simulink model "FAST"  (R2016a)
settings: Solver=FixedStepAuto  SolverMode=SingleTasking  StartTime=0.0  StopTime=600  FixedStep=DT  RelTol=1e-3
values from neighbouring files (symbols this model uses):
  delta_1p = (25*pi)/180    (= 0.436332312999)    [IPC_Control.m]
  delta_2p = (33*pi)/180    (= 0.575958653158)    [IPC_Control.m]
  IPC_Pitch_max = 5    [IPC_Control.m]
  k_1p = 1E-3    (= 0.001)    [IPC_Control.m]
  k_2p = 1E-3    (= 0.001)    [IPC_Control.m]
  ki_1p = 0.01    [IPC_Control.m]
  ki_2p = 0.002    [IPC_Control.m]
  omega_1p = (2*pi)/4.95    (= 1.26933036509)    [IPC_Control.m]
  omega_2p = (4*pi)/4.95    (= 2.53866073017)    [IPC_Control.m]
  omega_L = 10    [IPC_Control.m]
  zeta_1p = 0.5    [IPC_Control.m]
  zeta_2p = 0.3    [IPC_Control.m]
  zeta_L = 1    [IPC_Control.m]
undefined symbols (not defined in the file or in its folder): CertificationSettings, Control, DiscIntNeverNeededParam, dLP, Drivetrain, OutList, P_InitAngle, RPM_Init, strmatch, T_GenSpeedInit
settings Model: ExtModeTrigMode=oneshot  ExtModeArmWhenConnect=off  Creator=Hazim Namik  LastModifiedBy=jwvanwingerden
settings DataIOCC: LimitDataPoints=on  SaveFormat=Array
settings OptimizationCC: BlockReduction=off  BooleanDataType=off
settings DebuggingCC: SaveWithParameterizedLinksMsg=none  UnderspecifiedInitializationDetection=Classic  MergeDetectMultiDrivingBlocksExec=none  SignalResolutionControl=TryResolveAllWithWarning
settings HardwareCC: ProdBitPerPointer=32  ProdLargestAtomicFloat=None  ProdIntDivRoundTo=Undefined  ProdEndianess=Unspecified  ProdWordSize=32  ProdHWDeviceType=32-bit Generic  TargetUnknown=on
settings ModelReferenceCC: PropagateSignalLabelsOutOfModel=off

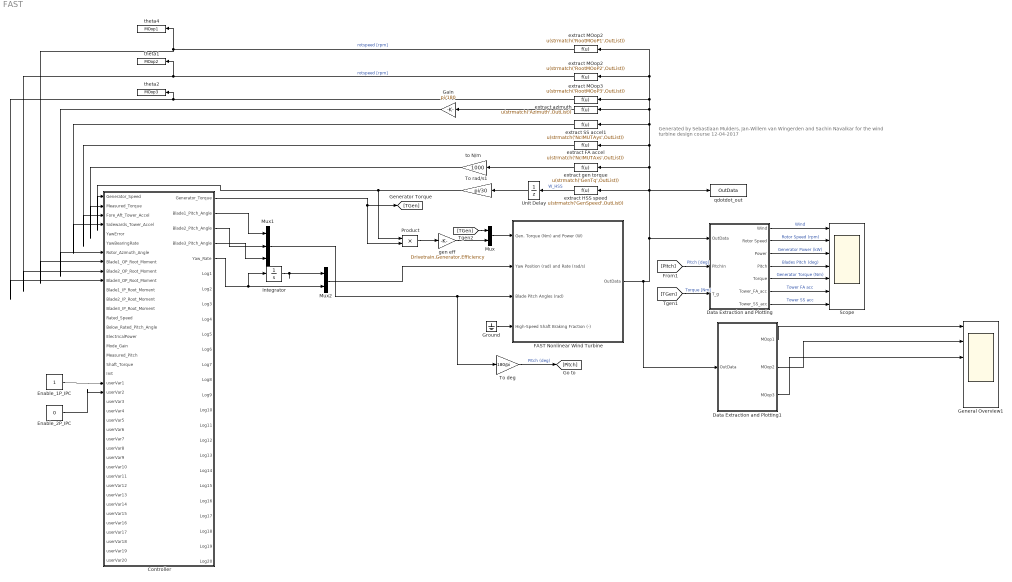
== system FAST ==
  note: Generated by Sebastiaan Mulders, Jan-Willem van Wingerden and Sachin Navalkar
      | for the wind turbine design course 12-04-2017
  Controller : Subsystem
  Data Extraction and Plotting : Subsystem
  Data Extraction and Plotting1 : Subsystem
  Enable_1P_IPC : Constant
  Enable_2P_IPC : Constant  Value=0
  FAST Nonlinear Wind Turbine : Subsystem  mask(FAST Nonlinear Wind Turbine){}
      mask help: This block contains the FAST S-Function.
      mask init:
      | clear FAST_SFunc
  Gain : Gain  Gain=pi/180
  General Overview1 : Scope  NumInputPorts=6
  Ground : Ground
  Integrator : Integrator
  Mux : Mux  Inputs=2
  Mux1 : Mux  Inputs=3
  Mux2 : Mux  Inputs=2
  Product : Product  RndMeth=Zero
  Scope : Scope  NumInputPorts=7
      settings: Tag=Scope
  To deg : Gain  Gain=180/pi
  To rad/s1 : Gain  Gain=pi/30
  Unit Delay : UnitDelay  InitialCondition=RPM_Init*Drivetrain.Gearbox.Ratio  SampleTime=-1
  extract FA accel : Fcn  Expr=u(strmatch('NcIMUTAxs',OutList))
  extract HSS speed : Fcn  Expr=u(strmatch('GenSpeed',OutList))
  extract MOop2 : Fcn  Expr=u(strmatch('RootMOoP2',OutList))
  "extract MOop2 " : Fcn  Expr=u(strmatch('RootMOoP1',OutList))
  extract MOop3 : Fcn  Expr=u(strmatch('RootMOoP3',OutList))
  extract SS accel1 : Fcn  Expr=u(strmatch('NcIMUTAys',OutList))
  extract azimuth : Fcn  Expr=u(strmatch('Azimuth',OutList))
  extract gen torque : Fcn  Expr=u(strmatch('GenTq',OutList))
  gen eff : Gain  Gain=Drivetrain.Generator.Efficiency
  qdotdot_out : ToWorkspace  VariableName=OutData  SampleTime=-1
  theta1 : ToWorkspace  VariableName=MOop2
      settings: MaxDataPoints=Inf
  theta2 : ToWorkspace  VariableName=MOop3
      settings: MaxDataPoints=Inf
  theta4 : ToWorkspace  VariableName=MOop1
      settings: MaxDataPoints=Inf
  to N/m : Gain  Gain=1000
  wires:
  Mux/1 -> FAST Nonlinear Wind Turbine/1(Gen. Torque (Nm) and Power (W))
  Mux2/1 -> FAST Nonlinear Wind Turbine/2(Yaw Position (rad) and Rate (rad/s))
  extract HSS speed/1 -> Unit Delay/1  "W_HSS"
  To deg/1 -> [Pitch]  "Pitch (deg)"
  gen eff/1 -> Mux/2
  Product/1 -> gen eff/1
  To rad/s1/1 -> Product/1, Controller/1(Generator_Speed)
  Data Extraction and Plotting/3(Power) -> Scope/3  "Generator Power (kW)"
  [Pitch] -> Data Extraction and Plotting/2(PitchIn)  "Pitch [deg]"
  Data Extraction and Plotting/1(Wind) -> Scope/1  "Wind"
  Data Extraction and Plotting/2(Rotor Speed) -> Scope/2  "Rotor Speed (rpm)"
  [TGen] -> Data Extraction and Plotting/3(T_g)  "Torque [Nm]"
  FAST Nonlinear Wind Turbine/1(OutData) -> Data Extraction and Plotting1/1(OutData), extract azimuth/1, extract MOop3/1, extract MOop2/1, "extract MOop2 "/1, extract SS accel1/1, extract FA accel/1, extract gen torque/1, extract HSS speed/1, qdotdot_out/1, Data Extraction and Plotting/1(OutData)
  Data Extraction and Plotting/4(Pitch) -> Scope/4  "Blades Pitch (deg)"
  Data Extraction and Plotting/5(Torque) -> Scope/5  "Generator Torque (Nm)"
  Unit Delay/1 -> To rad/s1/1
  extract gen torque/1 -> to N/m/1
  to N/m/1 -> Controller/2(Measured_Torque)
  Controller/1(Generator_Torque) -> Product/2, [TGen]
  extract FA accel/1 -> Controller/3(Fore_Aft_Tower_Accel)
  Data Extraction and Plotting/6(Tower_FA_acc) -> Scope/6  "Tower FA acc"
  Data Extraction and Plotting/7(Tower_SS_acc) -> Scope/7  "Tower SS acc"
  Ground/1 -> FAST Nonlinear Wind Turbine/4(High-Speed Shaft Braking Fraction (-))
  [TGen] -> Mux/1
  Mux1/1 -> To deg/1, FAST Nonlinear Wind Turbine/3(Blade Pitch Angles (rad))
  extract SS accel1/1 -> Controller/4(Sidewards_Tower_Accel)
  Controller/2(Blade1_Pitch_Angle) -> Mux1/1
  Controller/3(Blade2_Pitch_Angle) -> Mux1/2
  Controller/4(Blade3_Pitch_Angle) -> Mux1/3
  Integrator/1 -> Mux2/1
  Controller/5(Yaw_Rate) -> Integrator/1, Mux2/2
  "extract MOop2 "/1 -> theta4/1, Controller/8(Blade1_OP_Root_Moment)  "rotspeed [rpm]"
  extract MOop2/1 -> theta1/1, Controller/9(Blade2_OP_Root_Moment)  "rotspeed [rpm]"
  extract MOop3/1 -> Controller/10(Blade3_OP_Root_Moment), theta2/1
  Enable_1P_IPC/1 -> Controller/21(userVar1)
  Enable_2P_IPC/1 -> Controller/22(userVar2)
  extract azimuth/1 -> Gain/1
  Gain/1 -> Controller/7(Rotor_Azimuth_Angle)
  Data Extraction and Plotting1/1(MOop1) -> General Overview1/1
  Data Extraction and Plotting1/2(MOop2) -> General Overview1/2
  Data Extraction and Plotting1/3(MOop3) -> General Overview1/3

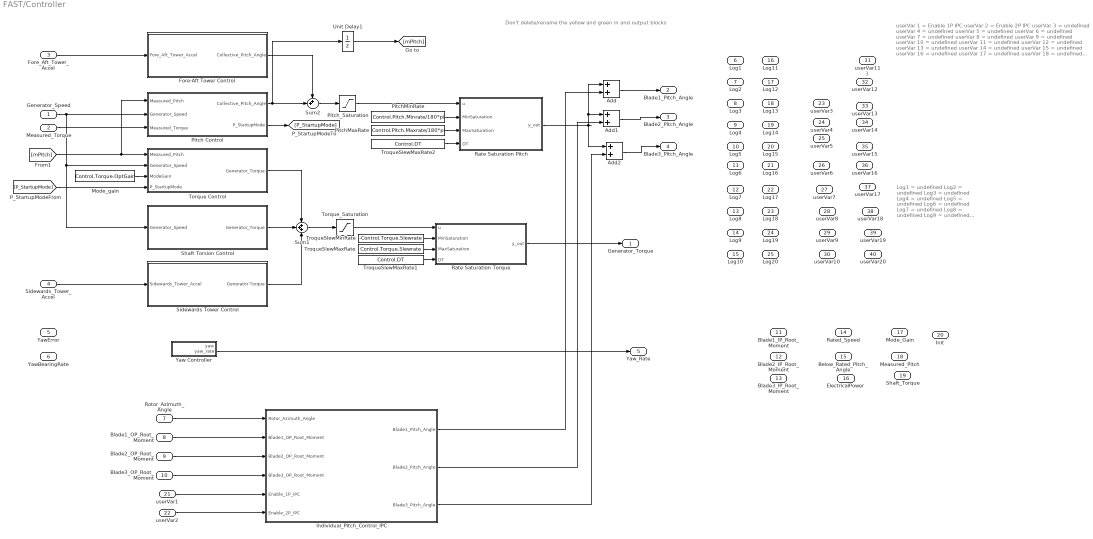
== system FAST/Controller ==
  note: Log1 		= 	undefined
      | Log2 		= 	undefined
      | Log3 		= 	undefined
      | Log4 		= 	undefined
      | Log5 		= 	undefined
      | Log6 		= 	undefined
      | Log7 		= 	undefined
      | Log8 		= 	undefined
      | Log9 		= 	undefined
      | Log10 		= 	undefined
      | Log11 		= 	undefined
      | Log12 		= 	undefined
      | Log13 		= 	undefined
      | Log14 		= 	undefined
      | Log15 		= 	undefined
      | Log16 		= 	undefined
      | Log17 		= 	undefined
      | Log18 		= 	undefined
      | Log19 		= 	undefined
      | Log20 		= 	undefined
  note: userVar 1 	=	Enable 1P IPC
      | userVar 2 	=	Enable 2P IPC
      | userVar 3 	=	undefined
      | userVar 4 	=	undefined
      | userVar 5 	=	undefined
      | userVar 6 	=	undefined
      | userVar 7 	=	undefined
      | userVar 8 	=	undefined
      | userVar 9 	=	undefined
      | userVar 10 	=	undefined
      | userVar 11 	=	undefined
      | userVar 12 	=	undefined
      | userVar 13 	=	undefined
      | userVar 14 	=	undefined
      | userVar 15 	=	undefined
      | userVar 16 	=	undefined
      | userVar 17 	=	undefined
      | userVar 18 	=	undefined
      | userVar 19 	=	undefined
      | userVar 20 	=	undefined
  note: Don't delete/rename the yellow and green in and output blocks
  note: 3
  Generator_Speed : Inport
  Measured_Torque : Inport  Port=2
  Fore_Aft_Tower_Accel : Inport  Port=3
  Sidewards_Tower_Accel : Inport  Port=4  PortDimensions=1
  YawError : Inport  Port=5  PortDimensions=1
  YawBearingRate : Inport  Port=6  PortDimensions=1
  Rotor_Azimuth_Angle : Inport  Port=7  PortDimensions=1
  Blade1_OP_Root_Moment : Inport  Port=8  PortDimensions=1
  Blade2_OP_Root_Moment : Inport  Port=9  PortDimensions=1
  Blade3_OP_Root_Moment : Inport  Port=10  PortDimensions=1
  Blade1_IP_Root_Moment : Inport  Port=11  PortDimensions=1
  Blade2_IP_Root_Moment : Inport  Port=12  PortDimensions=1
  Blade3_IP_Root_Moment : Inport  Port=13  PortDimensions=1
  Rated_Speed : Inport  Port=14  PortDimensions=1
  Below_Rated_Pitch_Angle : Inport  Port=15  PortDimensions=1
  ElectricalPower : Inport  Port=16  PortDimensions=1
  Mode_Gain : Inport  Port=17  PortDimensions=1
  Measured_Pitch : Inport  Port=18  PortDimensions=1
  Shaft_Torque : Inport  Port=19  PortDimensions=1
  Init : Inport  Port=20  PortDimensions=1
  userVar1 : Inport  Port=21  PortDimensions=1
  userVar2 : Inport  Port=22  PortDimensions=1
  userVar3 : Inport  Port=23  PortDimensions=1
  userVar4 : Inport  Port=24  PortDimensions=1
  userVar5 : Inport  Port=25  PortDimensions=1
  userVar6 : Inport  Port=26  PortDimensions=1
  userVar7 : Inport  Port=27  PortDimensions=1
  userVar8 : Inport  Port=28  PortDimensions=1
  userVar9 : Inport  Port=29  PortDimensions=1
  userVar10 : Inport  Port=30  PortDimensions=1
  userVar11 : Inport  Port=31  PortDimensions=1
  userVar12 : Inport  Port=32  PortDimensions=1
  userVar13 : Inport  Port=33  PortDimensions=1
  userVar14 : Inport  Port=34  PortDimensions=1
  userVar15 : Inport  Port=35  PortDimensions=1
  userVar16 : Inport  Port=36  PortDimensions=1
  userVar17 : Inport  Port=37  PortDimensions=1
  userVar18 : Inport  Port=38  PortDimensions=1
  userVar19 : Inport  Port=39  PortDimensions=1
  userVar20 : Inport  Port=40  PortDimensions=1
  Add : Sum
  Add1 : Sum
  Add2 : Sum
  Fore-Aft Tower Control : Subsystem
  Individual_Pitch_Control_IPC : Subsystem
  Mode_gain : Constant  Value=Control.Torque.OptGain
  Pitch Control : Subsystem
  PitchMaxRate : Constant  Value=Control.Pitch.Maxrate/180*pi
  PitchMinRate : Constant  Value=Control.Pitch.Minrate/180*pi
  Pitch_Saturation : Saturate  UpperLimit=Control.Pitch.Max*pi/180  LowerLimit=Control.Pitch.Min*pi/180
  Rate Saturation Pitch : MATLAB Function  TreatAsAtomicUnit=on
  Rate Saturation Torque : MATLAB Function  TreatAsAtomicUnit=on
  Shaft Torsion Control : Subsystem
  Sidewards Tower Control : Subsystem
  Sum1 : Sum  Inputs=+++
  Sum2 : Sum  Inputs=++|
  Torque Control : Subsystem
  Torque_Saturation : Saturate  UpperLimit=Control.Torque.Limit  LowerLimit=Control.Torque.Min
  TroqueSlewMaxRate : Constant  Value=Control.Torque.Slewrate
  TroqueSlewMaxRate1 : Constant  Value=Control.DT
  TroqueSlewMaxRate2 : Constant  Value=Control.DT
  TroqueSlewMinRate : Constant  Value=-Control.Torque.Slewrate
  Unit Delay1 : UnitDelay  InitialCondition=P_InitAngle*pi/180  SampleTime=-1
  Yaw Controller : Subsystem
  Generator_Torque : Outport
  Blade1_Pitch_Angle : Outport  Port=2  PortDimensions=1
  Blade2_Pitch_Angle : Outport  Port=3  PortDimensions=1
  Blade3_Pitch_Angle : Outport  Port=4  PortDimensions=1
  Yaw_Rate : Outport  Port=5  PortDimensions=1
  Log1 : Outport  Port=6  PortDimensions=1
  Log2 : Outport  Port=7  PortDimensions=1
  Log3 : Outport  Port=8  PortDimensions=1
  Log4 : Outport  Port=9  PortDimensions=1
  Log5 : Outport  Port=10  PortDimensions=1
  Log6 : Outport  Port=11  PortDimensions=1
  Log7 : Outport  Port=12  PortDimensions=1
  Log8 : Outport  Port=13  PortDimensions=1
  Log9 : Outport  Port=14  PortDimensions=1
  Log10 : Outport  Port=15  PortDimensions=1
  Log11 : Outport  Port=16  PortDimensions=1
  Log12 : Outport  Port=17  PortDimensions=1
  Log13 : Outport  Port=18  PortDimensions=1
  Log14 : Outport  Port=19  PortDimensions=1
  Log15 : Outport  Port=20  PortDimensions=1
  Log16 : Outport  Port=21  PortDimensions=1
  Log17 : Outport  Port=22  PortDimensions=1
  Log18 : Outport  Port=23  PortDimensions=1
  Log19 : Outport  Port=24  PortDimensions=1
  Log20 : Outport  Port=25  PortDimensions=1
  wires:
  Sidewards_Tower_Accel/1 -> Sidewards Tower Control/1(Sidewards_Tower_Accel)
  Fore_Aft_Tower_Accel/1 -> Fore-Aft Tower Control/1(Fore_Aft_Tower_Accel)
  Fore-Aft Tower Control/1(Collective_Pitch_Angle) -> Sum2/1
  Torque Control/1(Generator_Torque) -> Sum1/1
  Sidewards Tower Control/1(Generator Torque) -> Sum1/3
  [mPitch] -> Pitch Control/1(Measured_Pitch), Torque Control/1(Measured_Pitch)
  Measured_Torque/1 -> Pitch Control/3(Measured_Torque)
  Shaft Torsion Control/1(Generator_Torque) -> Sum1/2
  Mode_gain/1 -> Torque Control/3(ModeGain)
  Sum1/1 -> Torque_Saturation/1
  Unit Delay1/1 -> [mPitch]
  Sum2/1 -> Pitch_Saturation/1
  PitchMinRate/1 -> Rate Saturation Pitch/2(MinSaturation)
  PitchMaxRate/1 -> Rate Saturation Pitch/3(MaxSaturation)
  Pitch_Saturation/1 -> Rate Saturation Pitch/1(u)
  Torque_Saturation/1 -> Rate Saturation Torque/1(u)
  TroqueSlewMinRate/1 -> Rate Saturation Torque/2(MinSaturation)
  TroqueSlewMaxRate/1 -> Rate Saturation Torque/3(MaxSaturation)
  Generator_Speed/1 -> Pitch Control/2(Generator_Speed), Torque Control/2(Generator_Speed), Shaft Torsion Control/1(Generator_Speed)
  [P_StartupMode] -> Torque Control/4(P_StartupMode)
  Pitch Control/2(P_StartupMode) -> [P_StartupMode]
  Pitch Control/1(Collective_Pitch_Angle) -> Sum2/2, Unit Delay1/1
  Rate Saturation Torque/1(y_out) -> Generator_Torque/1
  TroqueSlewMaxRate1/1 -> Rate Saturation Torque/4(DT)
  TroqueSlewMaxRate2/1 -> Rate Saturation Pitch/4(DT)
  Rate Saturation Pitch/1(y_out) -> Add2/1, Add1/1, Add/1
  Yaw Controller/2(yaw_rate) -> Yaw_Rate/1
  Rotor_Azimuth_Angle/1 -> Individual_Pitch_Control_IPC/1(Rotor_Azimuth_Angle)
  Blade1_OP_Root_Moment/1 -> Individual_Pitch_Control_IPC/2(Blade1_OP_Root_Moment)
  Blade2_OP_Root_Moment/1 -> Individual_Pitch_Control_IPC/3(Blade2_OP_Root_Moment)
  Blade3_OP_Root_Moment/1 -> Individual_Pitch_Control_IPC/4(Blade3_OP_Root_Moment)
  userVar1/1 -> Individual_Pitch_Control_IPC/5(Enable_1P_IPC)
  userVar2/1 -> Individual_Pitch_Control_IPC/6(Enable_2P_IPC)
  Add/1 -> Blade1_Pitch_Angle/1
  Add1/1 -> Blade2_Pitch_Angle/1
  Add2/1 -> Blade3_Pitch_Angle/1
  Individual_Pitch_Control_IPC/1(Blade1_Pitch_Angle) -> Add/2
  Individual_Pitch_Control_IPC/2(Blade2_Pitch_Angle) -> Add1/2
  Individual_Pitch_Control_IPC/3(Blade3_Pitch_Angle) -> Add2/2

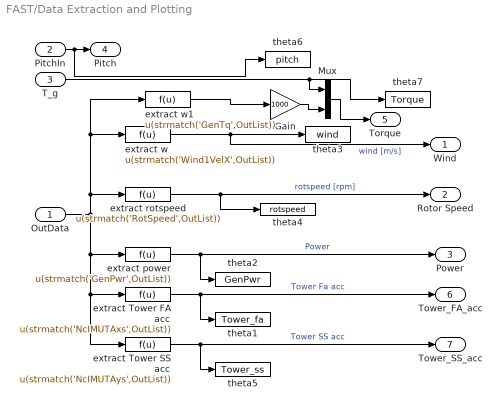
== system FAST/Data Extraction and Plotting ==
  OutData : Inport
  PitchIn : Inport  Port=2
  T_g : Inport  Port=3
  Gain : Gain  Gain=1000
  Mux : Mux  Inputs=2
  extract Tower FA acc : Fcn  Expr=u(strmatch('NcIMUTAxs',OutList))
  extract Tower SS acc : Fcn  Expr=u(strmatch('NcIMUTAys',OutList))
  extract power : Fcn  Expr=u(strmatch('GenPwr',OutList))
  extract rotspeed : Fcn  Expr=u(strmatch('RotSpeed',OutList))
  extract w : Fcn  Expr=u(strmatch('Wind1VelX',OutList))
  extract w1 : Fcn  Expr=u(strmatch('GenTq',OutList))
  theta1 : ToWorkspace  VariableName=Tower_fa  SampleTime=-1
      settings: MaxDataPoints=Inf  Decimation=3
  theta2 : ToWorkspace  VariableName=GenPwr  SampleTime=-1
      settings: MaxDataPoints=Inf  Decimation=3
  theta3 : ToWorkspace  VariableName=wind  SampleTime=-1
      settings: MaxDataPoints=Inf  Decimation=3
  theta4 : ToWorkspace  VariableName=rotspeed  SampleTime=-1
      settings: MaxDataPoints=Inf  Decimation=3
  theta5 : ToWorkspace  VariableName=Tower_ss  SampleTime=-1
      settings: MaxDataPoints=Inf  Decimation=3
  theta6 : ToWorkspace  VariableName=pitch  SampleTime=-1
      settings: MaxDataPoints=Inf  Decimation=3
  theta7 : ToWorkspace  VariableName=Torque  SampleTime=-1
      settings: MaxDataPoints=Inf  Decimation=3
  Wind : Outport
  Rotor Speed : Outport  Port=2
  Power : Outport  Port=3
  Pitch : Outport  Port=4
  Torque : Outport  Port=5
  Tower_FA_acc : Outport  Port=6
  Tower_SS_acc : Outport  Port=7
  wires:
  extract w/1 -> Wind/1, theta3/1  "wind [m/s]"
  extract rotspeed/1 -> theta4/1, Rotor Speed/1  "rotspeed [rpm]"
  extract power/1 -> theta2/1, Power/1  "Power"
  PitchIn/1 -> theta6/1, Pitch/1
  T_g/1 -> Mux/1, theta7/1
  extract Tower FA acc/1 -> theta1/1, Tower_FA_acc/1  "Tower Fa acc"
  OutData/1 -> extract w/1, extract w1/1, extract rotspeed/1, extract Tower SS acc/1, extract Tower FA acc/1, extract power/1
  extract Tower SS acc/1 -> theta5/1, Tower_SS_acc/1  "Tower SS acc"
  extract w1/1 -> Gain/1
  Gain/1 -> Mux/2
  Mux/1 -> Torque/1

== system FAST/Data Extraction and Plotting1 ==
  OutData : Inport
  "extract " : Fcn  Expr=u(strmatch('RootMOoP1',OutList))
  extract rotspeed1 : Fcn  Expr=u(strmatch('RootMOoP2',OutList))
  extract rotspeed2 : Fcn  Expr=u(strmatch('RootMOoP3',OutList))
  MOop1 : Outport
  MOop2 : Outport  Port=2
  MOop3 : Outport  Port=3
  wires:
  "extract "/1 -> MOop1/1  "rotspeed [rpm]"
  extract rotspeed1/1 -> MOop2/1  "rotspeed [rpm]"
  extract rotspeed2/1 -> MOop3/1  "rotspeed [rpm]"
  OutData/1 -> "extract "/1, extract rotspeed2/1, extract rotspeed1/1

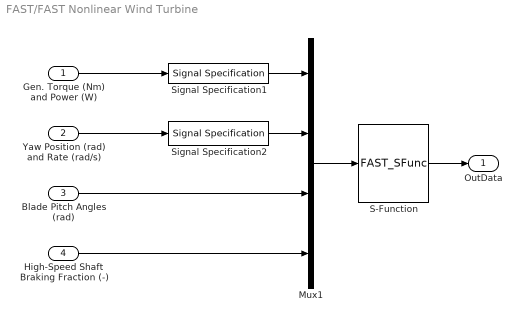
== system FAST/FAST Nonlinear Wind Turbine ==
  Gen. Torque (Nm) and Power (W) : Inport
  Yaw Position (rad) and Rate (rad/s) : Inport  Port=2
  Blade Pitch Angles (rad) : Inport  Port=3
  High-Speed Shaft Braking Fraction (-) : Inport  Port=4
  Mux1 : Mux
  S-Function : S-Function  FunctionName=FAST_SFunc  Parameters=FAST_InputFileName, TMax, 0  SFunctionDeploymentMode=off  EnableBusSupport=off
  Signal Specification1 : SignalSpecification  OutDataTypeStr=double  Dimensions=2
  Signal Specification2 : SignalSpecification  OutDataTypeStr=double  Dimensions=2
  OutData : Outport
  wires:
  Gen. Torque (Nm) and Power (W)/1 -> Signal Specification1/1
  S-Function/1 -> OutData/1
  Mux1/1 -> S-Function/1
  Blade Pitch Angles (rad)/1 -> Mux1/3
  Yaw Position (rad) and Rate (rad/s)/1 -> Signal Specification2/1
  Signal Specification1/1 -> Mux1/1
  Signal Specification2/1 -> Mux1/2
  High-Speed Shaft Braking Fraction (-)/1 -> Mux1/4

== system FAST/Controller/Fore-Aft Tower Control ==
  note: Fore-Aft tower damping
  Fore_Aft_Tower_Accel : Inport
  Discrete-Time Integrator : DiscreteIntegrator  SampleTime=-1  ICPrevOutput=DiscIntNeverNeededParam  ICPrevScaledInput=DiscIntNeverNeededParam
  Gain : Gain  Gain=Control.ForeAft.Gain
  Pitch_Saturation : Saturate  UpperLimit=Control.ForeAft.MaxPitchAmplitude*pi/180  LowerLimit=-Control.ForeAft.MaxPitchAmplitude*pi/180
  Collective_Pitch_Angle : Outport
  wires:
  Fore_Aft_Tower_Accel/1 -> Discrete-Time Integrator/1
  Pitch_Saturation/1 -> Collective_Pitch_Angle/1
  Discrete-Time Integrator/1 -> Gain/1
  Gain/1 -> Pitch_Saturation/1

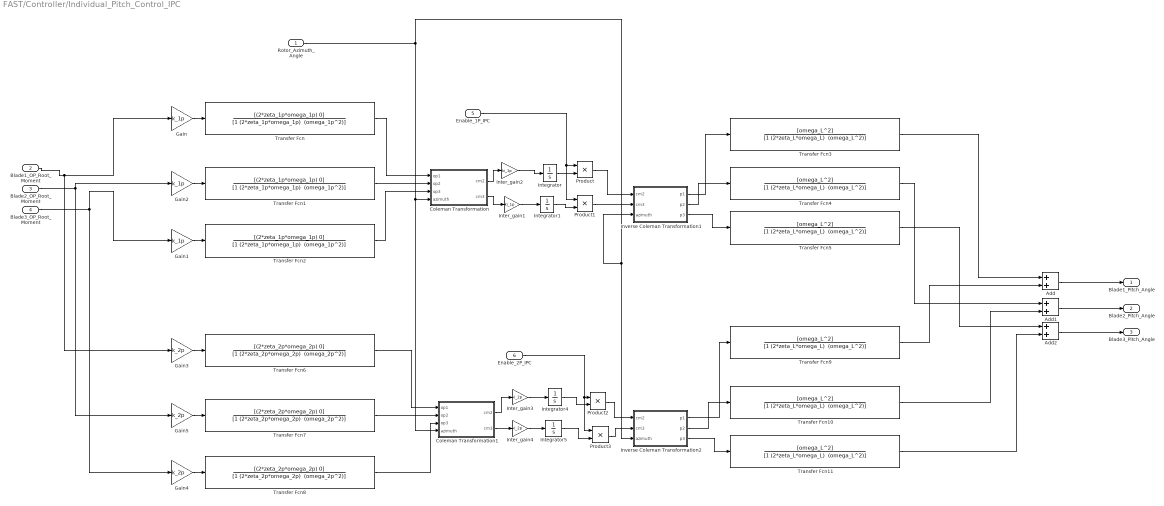
== system FAST/Controller/Individual_Pitch_Control_IPC ==
  Rotor_Azimuth_Angle : Inport
  Blade1_OP_Root_Moment : Inport  Port=2  PortDimensions=1
  Blade2_OP_Root_Moment : Inport  Port=3  PortDimensions=1
  Blade3_OP_Root_Moment : Inport  Port=4  PortDimensions=1
  Enable_1P_IPC : Inport  Port=5  PortDimensions=1
  Enable_2P_IPC : Inport  Port=6  PortDimensions=1
  Add : Sum
  Add1 : Sum
  Add2 : Sum
  Coleman Transformation : Subsystem
  Coleman Transformation1 : Subsystem
  Gain : Gain  Gain=k_1p
  Gain1 : Gain  Gain=k_1p
  Gain2 : Gain  Gain=k_1p
  Gain3 : Gain  Gain=k_2p
  Gain4 : Gain  Gain=k_2p
  Gain5 : Gain  Gain=k_2p
  Integrator{,1,4..5} (4 alike) : Integrator  LimitOutput=on  UpperSaturationLimit=IPC_Pitch_max*pi/180  LowerSaturationLimit=-IPC_Pitch_max*pi/180
  Inter_gain1 : Gain  Gain=ki_1p
  Inter_gain2 : Gain  Gain=ki_1p
  Inter_gain3 : Gain  Gain=ki_2p
  Inter_gain4 : Gain  Gain=ki_2p
  Inverse Coleman Transformation1 : Subsystem
  Inverse Coleman Transformation2 : Subsystem
  Product{,1..3} (4 alike) : Product
  Transfer Fcn : TransferFcn  Numerator=[(2*zeta_1p*omega_1p) 0]  Denominator="[1 (2*zeta_1p*omega_1p)  (omega_1p^2)]"
  Transfer Fcn1 : TransferFcn  Numerator=[(2*zeta_1p*omega_1p) 0]  Denominator="[1 (2*zeta_1p*omega_1p)  (omega_1p^2)]"
  Transfer Fcn{3..5,9..11} (6 alike) : TransferFcn  Numerator=[omega_L^2]  Denominator="[1 (2*zeta_L*omega_L)  (omega_L^2)]"
  Transfer Fcn2 : TransferFcn  Numerator=[(2*zeta_1p*omega_1p) 0]  Denominator="[1 (2*zeta_1p*omega_1p)  (omega_1p^2)]"
  Transfer Fcn6 : TransferFcn  Numerator=[(2*zeta_2p*omega_2p) 0]  Denominator="[1 (2*zeta_2p*omega_2p)  (omega_2p^2)]"
  Transfer Fcn7 : TransferFcn  Numerator=[(2*zeta_2p*omega_2p) 0]  Denominator="[1 (2*zeta_2p*omega_2p)  (omega_2p^2)]"
  Transfer Fcn8 : TransferFcn  Numerator=[(2*zeta_2p*omega_2p) 0]  Denominator="[1 (2*zeta_2p*omega_2p)  (omega_2p^2)]"
  Blade1_Pitch_Angle : Outport  PortDimensions=1
  Blade2_Pitch_Angle : Outport  Port=2  PortDimensions=1
  Blade3_Pitch_Angle : Outport  Port=3  PortDimensions=1
  wires:
  Rotor_Azimuth_Angle/1 -> Inverse Coleman Transformation1/3(azimuth), Inverse Coleman Transformation2/3(azimuth), Coleman Transformation1/4(azimuth), Coleman Transformation/4(azimuth)
  Coleman Transformation/1(cm2) -> Inter_gain2/1
  Coleman Transformation/2(cm3) -> Inter_gain1/1
  Inter_gain1/1 -> Integrator1/1
  Gain/1 -> Transfer Fcn/1
  Transfer Fcn/1 -> Coleman Transformation/1(op1)
  Gain1/1 -> Transfer Fcn2/1
  Transfer Fcn2/1 -> Coleman Transformation/3(op3)
  Gain2/1 -> Transfer Fcn1/1
  Transfer Fcn1/1 -> Coleman Transformation/2(op2)
  Inverse Coleman Transformation1/1(p1) -> Transfer Fcn3/1
  Inverse Coleman Transformation1/2(p2) -> Transfer Fcn4/1
  Inverse Coleman Transformation1/3(p3) -> Transfer Fcn5/1
  Blade1_OP_Root_Moment/1 -> Gain3/1, Gain/1
  Blade3_OP_Root_Moment/1 -> Gain1/1, Gain4/1
  Blade2_OP_Root_Moment/1 -> Gain2/1, Gain5/1
  Gain3/1 -> Transfer Fcn6/1
  Gain4/1 -> Transfer Fcn8/1
  Gain5/1 -> Transfer Fcn7/1
  Transfer Fcn6/1 -> Coleman Transformation1/1(op1)
  Transfer Fcn7/1 -> Coleman Transformation1/2(op2)
  Transfer Fcn8/1 -> Coleman Transformation1/3(op3)
  Coleman Transformation1/1(cm2) -> Inter_gain3/1
  Coleman Transformation1/2(cm3) -> Inter_gain4/1
  Inverse Coleman Transformation2/1(p1) -> Transfer Fcn9/1
  Inverse Coleman Transformation2/2(p2) -> Transfer Fcn10/1
  Inverse Coleman Transformation2/3(p3) -> Transfer Fcn11/1
  Transfer Fcn4/1 -> Add1/1
  Transfer Fcn5/1 -> Add2/1
  Transfer Fcn9/1 -> Add/2
  Transfer Fcn10/1 -> Add1/2
  Transfer Fcn11/1 -> Add2/2
  Add/1 -> Blade1_Pitch_Angle/1
  Add1/1 -> Blade2_Pitch_Angle/1
  Add2/1 -> Blade3_Pitch_Angle/1
  Inter_gain2/1 -> Integrator/1
  Transfer Fcn3/1 -> Add/1
  Inter_gain3/1 -> Integrator4/1
  Inter_gain4/1 -> Integrator5/1
  Integrator/1 -> Product/2
  Product/1 -> Inverse Coleman Transformation1/1(cm2)
  Enable_1P_IPC/1 -> Product1/1, Product/1
  Integrator1/1 -> Product1/2
  Product1/1 -> Inverse Coleman Transformation1/2(cm3)
  Enable_2P_IPC/1 -> Product3/1, Product2/1
  Integrator4/1 -> Product2/2
  Product2/1 -> Inverse Coleman Transformation2/1(cm2)
  Integrator5/1 -> Product3/2
  Product3/1 -> Inverse Coleman Transformation2/2(cm3)

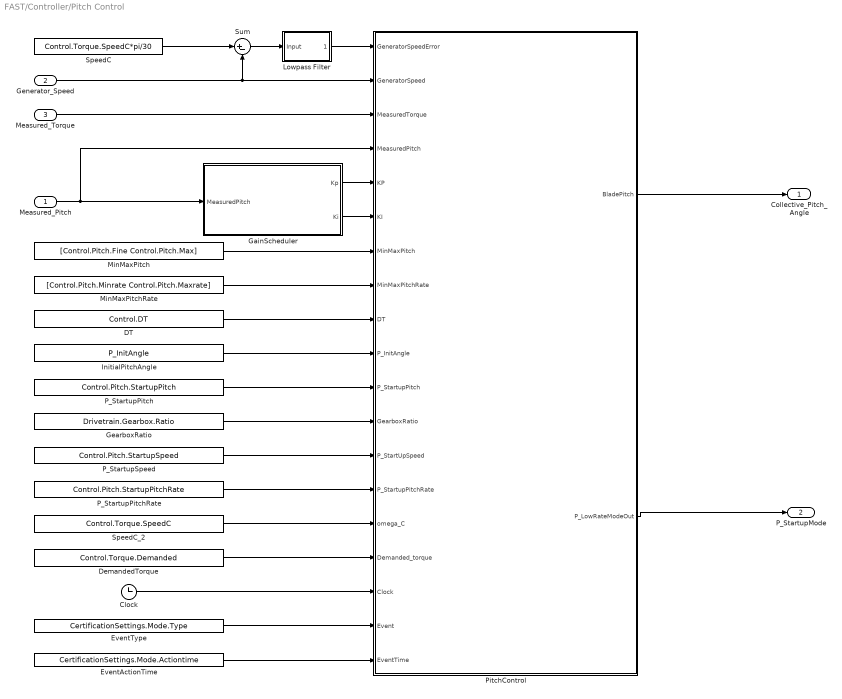
== system FAST/Controller/Pitch Control ==
  Measured_Pitch : Inport
  Generator_Speed : Inport  Port=2
  Measured_Torque : Inport  Port=3
  Clock : Clock
  DT : Constant  Value=Control.DT
  DemandedTorque : Constant  Value=Control.Torque.Demanded
  EventActionTime : Constant  Value=CertificationSettings.Mode.Actiontime
  EventType : Constant  Value=CertificationSettings.Mode.Type
  GainScheduler : Subsystem
  GearboxRatio : Constant  Value=Drivetrain.Gearbox.Ratio
  InitialPitchAngle : Constant  Value=P_InitAngle
  Lowpass Filter : Subsystem
  MinMaxPitch : Constant  Value=[Control.Pitch.Fine Control.Pitch.Max]
  MinMaxPitchRate : Constant  Value=[Control.Pitch.Minrate Control.Pitch.Maxrate]
  P_StartupPitch : Constant  Value=Control.Pitch.StartupPitch
  P_StartupPitchRate : Constant  Value=Control.Pitch.StartupPitchRate
  P_StartupSpeed : Constant  Value=Control.Pitch.StartupSpeed
  PitchControl : MATLAB Function  TreatAsAtomicUnit=on
  SpeedC : Constant  Value=Control.Torque.SpeedC*pi/30
  SpeedC_2 : Constant  Value=Control.Torque.SpeedC
  Sum : Sum  Inputs=|+-
  Collective_Pitch_Angle : Outport
  P_StartupMode : Outport  Port=2
  wires:
  MinMaxPitch/1 -> PitchControl/7(MinMaxPitch)
  MinMaxPitchRate/1 -> PitchControl/8(MinMaxPitchRate)
  PitchControl/1(BladePitch) -> Collective_Pitch_Angle/1
  Measured_Torque/1 -> PitchControl/3(MeasuredTorque)
  SpeedC/1 -> Sum/1
  Generator_Speed/1 -> PitchControl/2(GeneratorSpeed), Sum/2
  Sum/1 -> Lowpass Filter/1(Input)
  Lowpass Filter/1(Output) -> PitchControl/1(GeneratorSpeedError)
  PitchControl/2(P_LowRateModeOut) -> P_StartupMode/1
  DT/1 -> PitchControl/9(DT)
  P_StartupPitch/1 -> PitchControl/11(P_StartupPitch)
  InitialPitchAngle/1 -> PitchControl/10(P_InitAngle)
  GearboxRatio/1 -> PitchControl/12(GearboxRatio)
  P_StartupSpeed/1 -> PitchControl/13(P_StartUpSpeed)
  P_StartupPitchRate/1 -> PitchControl/14(P_StartupPitchRate)
  SpeedC_2/1 -> PitchControl/15(omega_C)
  DemandedTorque/1 -> PitchControl/16(Demanded_torque)
  Measured_Pitch/1 -> PitchControl/4(MeasuredPitch), GainScheduler/1(MeasuredPitch)
  EventType/1 -> PitchControl/18(Event)
  Clock/1 -> PitchControl/17(Clock)
  EventActionTime/1 -> PitchControl/19(EventTime)
  GainScheduler/1(Kp) -> PitchControl/5(KP)
  GainScheduler/2(Ki) -> PitchControl/6(KI)

== system FAST/Controller/Shaft Torsion Control ==
  Generator_Speed : Inport
  Gain : Gain  Gain=0
  Generator_Torque : Outport
  wires:
  Generator_Speed/1 -> Gain/1
  Gain/1 -> Generator_Torque/1

== system FAST/Controller/Sidewards Tower Control ==
  Sidewards_Tower_Accel : Inport
  Gain : Gain  Gain=0
  Generator Torque : Outport
  wires:
  Sidewards_Tower_Accel/1 -> Gain/1
  Gain/1 -> Generator Torque/1

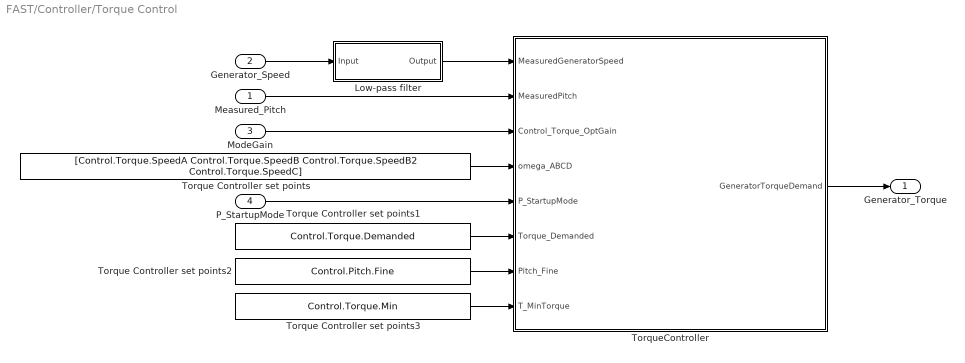
== system FAST/Controller/Torque Control ==
  Measured_Pitch : Inport
  Generator_Speed : Inport  Port=2
  ModeGain : Inport  Port=3
  P_StartupMode : Inport  Port=4
  Low-pass filter : Subsystem
  Torque Controller set points : Constant  Value=[Control.Torque.SpeedA Control.Torque.SpeedB Control.Torque.SpeedB2 Control.Torque.SpeedC]
  Torque Controller set points1 : Constant  Value=Control.Torque.Demanded
  Torque Controller set points2 : Constant  Value=Control.Pitch.Fine
  Torque Controller set points3 : Constant  Value=Control.Torque.Min
  TorqueController : MATLAB Function  TreatAsAtomicUnit=on
  Generator_Torque : Outport
  wires:
  Generator_Speed/1 -> Low-pass filter/1(Input)
  TorqueController/1(GeneratorTorqueDemand) -> Generator_Torque/1
  Measured_Pitch/1 -> TorqueController/2(MeasuredPitch)
  ModeGain/1 -> TorqueController/3(Control_Torque_OptGain)
  Torque Controller set points/1 -> TorqueController/4(omega_ABCD)
  P_StartupMode/1 -> TorqueController/5(P_StartupMode)
  Low-pass filter/1(Output) -> TorqueController/1(MeasuredGeneratorSpeed)
  Torque Controller set points3/1 -> TorqueController/8(T_MinTorque)
  Torque Controller set points2/1 -> TorqueController/7(Pitch_Fine)
  Torque Controller set points1/1 -> TorqueController/6(Torque_Demanded)

== system FAST/Controller/Yaw Controller ==
  Yaw Position : Constant  Value=0
  Yaw rate : Constant  Value=0
  yaw : Outport
  yaw_rate : Outport  Port=2
  wires:
  Yaw Position/1 -> yaw/1
  Yaw rate/1 -> yaw_rate/1

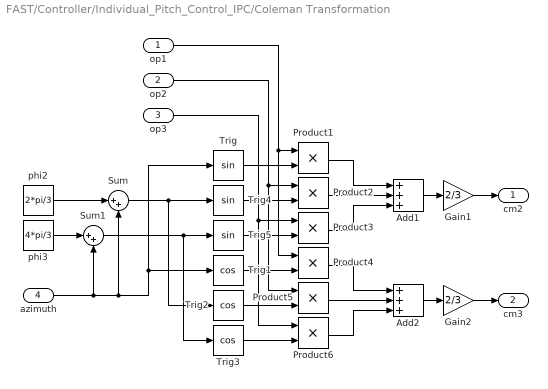
== system FAST/Controller/Individual_Pitch_Control_IPC/Coleman Transformation ==
  op1 : Inport
  op2 : Inport  Port=2
  op3 : Inport  Port=3
  azimuth : Inport  Port=4
  Add1 : Sum  Inputs=+++
  Add2 : Sum  Inputs=+++
  Gain1 : Gain  Gain=2/3
  Gain2 : Gain  Gain=2/3
  Product{1..6} (6 alike) : Product  RndMeth=Zero
  Sum : Sum  Inputs=|++
  Sum1 : Sum  Inputs=|++
  Trig : Trigonometry
  Trig1 : Trigonometry  Operator=cos
  Trig2 : Trigonometry  Operator=cos
  Trig3 : Trigonometry  Operator=cos
  Trig4 : Trigonometry
  Trig5 : Trigonometry
  phi2 : Constant  Value=2*pi/3
  phi3 : Constant  Value=4*pi/3
  cm2 : Outport
  cm3 : Outport  Port=2
  wires:
  Add1/1 -> Gain1/1
  phi2/1 -> Sum/1
  phi3/1 -> Sum1/1
  azimuth/1 -> Sum1/2, Sum/2, Trig/1, Trig1/1
  Trig/1 -> Product1/2
  Trig4/1 -> Product2/2
  Trig5/1 -> Product3/2
  Trig1/1 -> Product4/2
  Trig2/1 -> Product5/2
  Trig3/1 -> Product6/2
  Sum/1 -> Trig4/1, Trig2/1
  Sum1/1 -> Trig5/1, Trig3/1
  Add2/1 -> Gain2/1
  Gain1/1 -> cm2/1
  Gain2/1 -> cm3/1
  op1/1 -> Product1/1, Product4/1
  op2/1 -> Product2/1, Product5/1
  op3/1 -> Product6/1, Product3/1
  Product1/1 -> Add1/1
  Product2/1 -> Add1/2
  Product3/1 -> Add1/3
  Product4/1 -> Add2/1
  Product5/1 -> Add2/2
  Product6/1 -> Add2/3

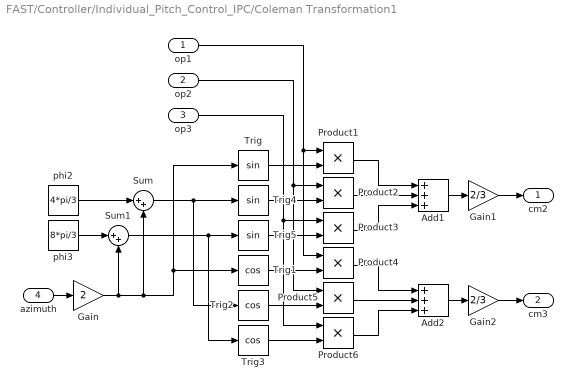
== system FAST/Controller/Individual_Pitch_Control_IPC/Coleman Transformation1 ==
  op1 : Inport
  op2 : Inport  Port=2
  op3 : Inport  Port=3
  azimuth : Inport  Port=4
  Add1 : Sum  Inputs=+++
  Add2 : Sum  Inputs=+++
  Gain : Gain  Gain=2
  Gain1 : Gain  Gain=2/3
  Gain2 : Gain  Gain=2/3
  Product{1..6} (6 alike) : Product  RndMeth=Zero
  Sum : Sum  Inputs=|++
  Sum1 : Sum  Inputs=|++
  Trig : Trigonometry
  Trig1 : Trigonometry  Operator=cos
  Trig2 : Trigonometry  Operator=cos
  Trig3 : Trigonometry  Operator=cos
  Trig4 : Trigonometry
  Trig5 : Trigonometry
  phi2 : Constant  Value=4*pi/3
  phi3 : Constant  Value=8*pi/3
  cm2 : Outport
  cm3 : Outport  Port=2
  wires:
  Add1/1 -> Gain1/1
  phi2/1 -> Sum/1
  phi3/1 -> Sum1/1
  azimuth/1 -> Gain/1
  Trig/1 -> Product1/2
  Trig4/1 -> Product2/2
  Trig5/1 -> Product3/2
  Trig1/1 -> Product4/2
  Trig2/1 -> Product5/2
  Trig3/1 -> Product6/2
  Sum/1 -> Trig4/1, Trig2/1
  Sum1/1 -> Trig5/1, Trig3/1
  Add2/1 -> Gain2/1
  Gain1/1 -> cm2/1
  Gain2/1 -> cm3/1
  op1/1 -> Product1/1, Product4/1
  op2/1 -> Product2/1, Product5/1
  op3/1 -> Product6/1, Product3/1
  Product1/1 -> Add1/1
  Product2/1 -> Add1/2
  Product3/1 -> Add1/3
  Product4/1 -> Add2/1
  Product5/1 -> Add2/2
  Product6/1 -> Add2/3
  Gain/1 -> Sum1/2, Sum/2, Trig/1, Trig1/1

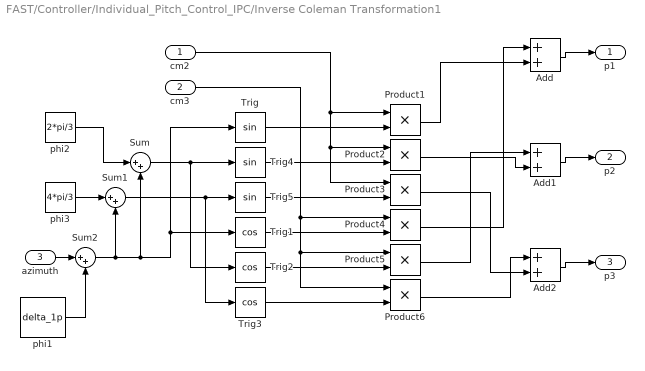
== system FAST/Controller/Individual_Pitch_Control_IPC/Inverse Coleman Transformation1 ==
  cm2 : Inport
  cm3 : Inport  Port=2
  azimuth : Inport  Port=3
  Add : Sum
  Add1 : Sum
  Add2 : Sum
  Product{1..6} (6 alike) : Product  RndMeth=Zero
  Sum : Sum  Inputs=|++
  Sum1 : Sum  Inputs=|++
  Sum2 : Sum  Inputs=|++
  Trig : Trigonometry
  Trig1 : Trigonometry  Operator=cos
  Trig2 : Trigonometry  Operator=cos
  Trig3 : Trigonometry  Operator=cos
  Trig4 : Trigonometry
  Trig5 : Trigonometry
  phi1 : Constant  Value=delta_1p
  phi2 : Constant  Value=2*pi/3
  phi3 : Constant  Value=4*pi/3
  p1 : Outport
  p2 : Outport  Port=2
  p3 : Outport  Port=3
  wires:
  phi2/1 -> Sum/1
  phi3/1 -> Sum1/1
  Sum2/1 -> Sum1/2, Sum/2, Trig/1, Trig1/1
  Sum/1 -> Trig4/1, Trig2/1
  Sum1/1 -> Trig5/1, Trig3/1
  Add/1 -> p1/1
  Add1/1 -> p2/1
  Add2/1 -> p3/1
  Trig/1 -> Product1/2
  Trig4/1 -> Product2/2
  Trig5/1 -> Product3/2
  Trig1/1 -> Product4/2
  Trig2/1 -> Product5/2
  Trig3/1 -> Product6/2
  cm2/1 -> Product1/1, Product2/1, Product3/1
  Product1/1 -> Add/2
  Product2/1 -> Add1/2
  Product3/1 -> Add2/2
  cm3/1 -> Product4/1, Product5/1, Product6/1
  Product4/1 -> Add/1
  Product5/1 -> Add1/1
  Product6/1 -> Add2/1
  phi1/1 -> Sum2/2
  azimuth/1 -> Sum2/1

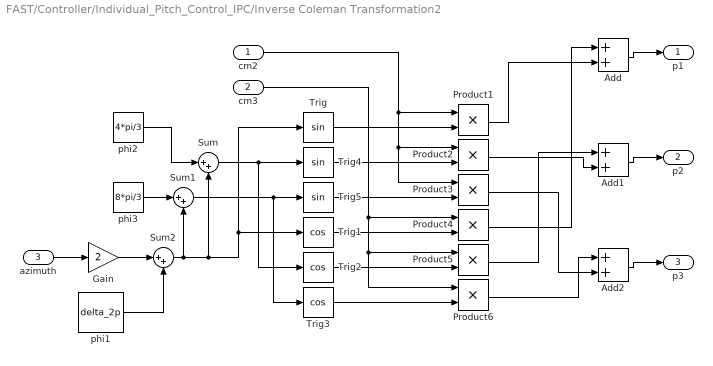
== system FAST/Controller/Individual_Pitch_Control_IPC/Inverse Coleman Transformation2 ==
  cm2 : Inport
  cm3 : Inport  Port=2
  azimuth : Inport  Port=3
  Add : Sum
  Add1 : Sum
  Add2 : Sum
  Gain : Gain  Gain=2
  Product{1..6} (6 alike) : Product  RndMeth=Zero
  Sum : Sum  Inputs=|++
  Sum1 : Sum  Inputs=|++
  Sum2 : Sum  Inputs=|++
  Trig : Trigonometry
  Trig1 : Trigonometry  Operator=cos
  Trig2 : Trigonometry  Operator=cos
  Trig3 : Trigonometry  Operator=cos
  Trig4 : Trigonometry
  Trig5 : Trigonometry
  phi1 : Constant  Value=delta_2p
  phi2 : Constant  Value=4*pi/3
  phi3 : Constant  Value=8*pi/3
  p1 : Outport
  p2 : Outport  Port=2
  p3 : Outport  Port=3
  wires:
  phi2/1 -> Sum/1
  phi3/1 -> Sum1/1
  Sum2/1 -> Sum/2, Trig/1, Trig1/1, Sum1/2
  Sum/1 -> Trig4/1, Trig2/1
  Sum1/1 -> Trig5/1, Trig3/1
  Add/1 -> p1/1
  Add1/1 -> p2/1
  Add2/1 -> p3/1
  Trig/1 -> Product1/2
  Trig4/1 -> Product2/2
  Trig5/1 -> Product3/2
  Trig1/1 -> Product4/2
  Trig2/1 -> Product5/2
  Trig3/1 -> Product6/2
  cm2/1 -> Product1/1, Product2/1, Product3/1
  Product1/1 -> Add/2
  Product2/1 -> Add1/2
  Product3/1 -> Add2/2
  cm3/1 -> Product4/1, Product5/1, Product6/1
  Product4/1 -> Add/1
  Product5/1 -> Add1/1
  Product6/1 -> Add2/1
  azimuth/1 -> Gain/1
  phi1/1 -> Sum2/2
  Gain/1 -> Sum2/1

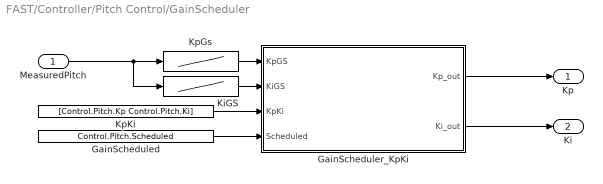
== system FAST/Controller/Pitch Control/GainScheduler ==
  MeasuredPitch : Inport
  GainScheduled : Constant  Value=Control.Pitch.Scheduled
  GainScheduler_KpKi : MATLAB Function  TreatAsAtomicUnit=on
  KiGS : Lookup_n-D  NumberOfTableDimensions=1  BreakpointsForDimension1=Control.Pitch.ScheduledPitchAngles  Table=Control.Pitch.KiGS  ExtrapMethod=Clip  UseLastTableValue=on  InternalRulePriority=Speed  RndMeth=Simplest  InputSameDT=on
  KpGs : Lookup_n-D  NumberOfTableDimensions=1  BreakpointsForDimension1=Control.Pitch.ScheduledPitchAngles  Table=Control.Pitch.KpGS  ExtrapMethod=Clip  UseLastTableValue=on  InternalRulePriority=Speed  RndMeth=Simplest  InputSameDT=on
  KpKi : Constant  Value=[Control.Pitch.Kp Control.Pitch.Ki]
  Kp : Outport
  Ki : Outport  Port=2
  wires:
  MeasuredPitch/1 -> KiGS/1, KpGs/1
  GainScheduled/1 -> GainScheduler_KpKi/4(Scheduled)
  GainScheduler_KpKi/2(Ki_out) -> Ki/1
  KpKi/1 -> GainScheduler_KpKi/3(KpKi)
  KpGs/1 -> GainScheduler_KpKi/1(KpGS)
  KiGS/1 -> GainScheduler_KpKi/2(KiGS)
  GainScheduler_KpKi/1(Kp_out) -> Kp/1

== system FAST/Controller/Pitch Control/Lowpass Filter ==
  Input : Inport
  Discrete State-Space : DiscreteStateSpace  A=dLP.a  B=dLP.b  C=dLP.c  D=dLP.d  SampleTime=-1
  Output : Outport
  wires:
  Input/1 -> Discrete State-Space/1
  Discrete State-Space/1 -> Output/1

== system FAST/Controller/Torque Control/Low-pass filter ==
  Input : Inport
  Low-pass filter : DiscreteStateSpace  A=dLP.a  B=dLP.b  C=dLP.c  D=dLP.d  X0=T_GenSpeedInit*(pi/30)/dLP.c  SampleTime=-1
  Output : Outport
  wires:
  Input/1 -> Low-pass filter/1
  Low-pass filter/1 -> Output/1

== matlab function FAST/Controller/Rate Saturation Torque ==
  data: u input; MinSaturation input; y_out output; MaxSaturation input; DT input
function y_out = fcn(u, MinSaturation, MaxSaturation, DT)
persistent y

if isempty(y)
    y = u;
end

rate = (u-y)/DT;
rate = min(max(rate, MinSaturation), MaxSaturation);

y = y + rate*DT;
y_out = y;

== matlab function FAST/Controller/Rate Saturation Pitch ==
  data: u input; MinSaturation input; y_out output; MaxSaturation input; DT input
function y_out = fcn(u, MinSaturation, MaxSaturation, DT)
persistent y

if isempty(y)
    y = u;
end

rate = (u-y)/DT;
rate = min(max(rate, MinSaturation), MaxSaturation);

y = y + rate*DT;
y_out = y;

== matlab function FAST/Controller/Torque Control/TorqueController ==
  data: GeneratorTorqueDemand output; MeasuredGeneratorSpeed input; MeasuredPitch input; Control_Torque_OptGain input; omega_ABCD input size=[1 4]; P_StartupMode input; Torque_Demanded input; Pitch_Fine input; T_MinTorque input
function GeneratorTorqueDemand  = TorqueController(MeasuredGeneratorSpeed, MeasuredPitch, Control_Torque_OptGain, omega_ABCD, P_StartupMode, Torque_Demanded, Pitch_Fine, T_MinTorque)

% Calculate generator torque setpoint according to the feedforward wind
% turbine control law T = K*\omega^2
GeneratorTorqueDemand = max(min(Control_Torque_OptGain*MeasuredGeneratorSpeed^2, Torque_Demanded), T_MinTorque);

% Calculate torques at beginning and end of CP_max operation
TorqueOmegaB = Control_Torque_OptGain*(omega_ABCD(2)*pi/30)^2;
TorqueOmegaC = Control_Torque_OptGain*(omega_ABCD(3)*pi/30)^2;

% Apply maximum demanded torque when pitch is 1 degree above fine-pitch and
% the wind turbine is not in start-up mode.
if MeasuredPitch > (Pitch_Fine + 1)*pi/180 && P_StartupMode == false
    GeneratorTorqueDemand = Torque_Demanded;
elseif MeasuredGeneratorSpeed < omega_ABCD(1)*pi/30
    GeneratorTorqueDemand = T_MinTorque;
elseif MeasuredGeneratorSpeed < omega_ABCD(2)*pi/30
    GeneratorTorqueDemand = (TorqueOmegaB - T_MinTorque)/((omega_ABCD(2) - omega_ABCD(1))*pi/30)*(MeasuredGeneratorSpeed - omega_ABCD(1)*pi/30) + T_MinTorque;
elseif MeasuredGeneratorSpeed >= omega_ABCD(3)*pi/30
    GeneratorTorqueDemand = (Torque_Demanded - TorqueOmegaC)/((omega_ABCD(4) - omega_ABCD(3))*pi/30)*(MeasuredGeneratorSpeed - omega_ABCD(3)*pi/30) + TorqueOmegaC;
end

== matlab function FAST/Controller/Pitch Control/PitchControl ==
  settings: updateMethod=DISCRETE  sampleTime=DT
  data: GeneratorSpeedError input; GeneratorSpeed input; MeasuredTorque input; MeasuredPitch input; BladePitch output; KP input; KI input; MinMaxPitch input; MinMaxPitchRate input; DT input; P_InitAngle input; P_StartupPitch input; GearboxRatio input; P_StartUpSpeed input; P_StartupPitchRate input; omega_C input; Demanded_torque input; Clock input; P_LowRateModeOut output; Event input; EventTime input
function [BladePitch, P_LowRateModeOut]  = PitchControl(GeneratorSpeedError, GeneratorSpeed, MeasuredTorque, MeasuredPitch, KP, KI, MinMaxPitch, MinMaxPitchRate, DT, P_InitAngle, P_StartupPitch, GearboxRatio, P_StartUpSpeed, P_StartupPitchRate, omega_C, Demanded_torque, Clock, Event, EventTime)
persistent I_term PI_term_old P_LowRateMode P_LowRateMode_old

%Initialize all persistent variables
if isempty(I_term)
    I_term = (P_InitAngle*pi/180);
    PI_term_old = (P_InitAngle*pi/180);
    P_LowRateMode = true;
    P_LowRateMode_old = true; %Used to detect change from start-up/below-rated to above-rated operation mode
end

%Event handling part
if (Event == 2 && Clock >= EventTime) || (Event == 5 && Clock >= EventTime) %Grid loss, emergency shutdown
    P_LowRateMode = false;
    P_MinPitchSat = MinMaxPitch(2)*pi/180;
elseif (Event == 4 && Clock >= EventTime) % Normal shutdown
    P_LowRateMode = true;
    P_MinPitchSat = MinMaxPitch(2)*pi/180;
elseif Event == 7 || Event == 6 % Idling and parked mode
    P_MinPitchSat = MinMaxPitch(2)*pi/180;
elseif MeasuredTorque > Demanded_torque*0.99 || GeneratorSpeed > omega_C*(pi/30) % Above-rated operating mode
    P_LowRateMode = false;
    P_MinPitchSat = MinMaxPitch(1)*pi/180;
    if P_LowRateMode ~= P_LowRateMode_old % On switching event between below-rated to above rated, reinitialize the integral term to ensure smooth transition
        I_term = MeasuredPitch;
    end
elseif Event == 3 || GeneratorSpeed < P_StartUpSpeed*GearboxRatio*(pi/30) % Normal startup 
    if Event == 3 && Clock < EventTime
        P_LowRateMode = true;
        P_MinPitchSat = MinMaxPitch(2)*pi/180;
    elseif (Event == 3 && Clock >= EventTime) && (GeneratorSpeed < P_StartUpSpeed*GearboxRatio*(pi/30))
        P_LowRateMode = true;
        P_MinPitchSat = P_StartupPitch*pi/180;
    else
        P_LowRateMode = true;
        P_MinPitchSat = MinMaxPitch(1)*pi/180;
    end
else
    P_MinPitchSat = MinMaxPitch(1)*pi/180;
end
 
% Pitch controller, KP and KI are constant or gain-scheduled, depending on
% input. Integral term is saturated, lower bound is variable and depends on
% event or operatinig mode.
P_term = KP*GeneratorSpeedError;
I_term = I_term + KI*GeneratorSpeedError*DT;
I_term = min(max(I_term,P_MinPitchSat), MinMaxPitch(2)*pi/180);

PI_term = P_term + I_term;
PI_term_sat = min(max(PI_term,P_MinPitchSat), MinMaxPitch(2)*pi/180);

% Calculate and limit pitch rate. Limit on rate is subject to event or
% operating mode.
PitchRate = (PI_term_sat - PI_term_old)/DT;
if P_LowRateMode
    PitchRate = min(max(PitchRate, -P_StartupPitchRate*pi/180), P_StartupPitchRate*pi/180);
else
    PitchRate = min(max(PitchRate, MinMaxPitchRate(1)*pi/180), MinMaxPitchRate(2)*pi/180);
end
BladePitch = PI_term_old + PitchRate*DT;

% Write variables to persistent variables and/or outputs
PI_term_old = BladePitch;
P_LowRateModeOut = P_LowRateMode;
P_LowRateMode_old = P_LowRateMode;
end

== matlab function FAST/Controller/Pitch Control/GainScheduler/GainScheduler_KpKi ==
  data: KpGS input; KiGS input; Kp_out output; KpKi input; Scheduled input; Ki_out output
function [Kp_out, Ki_out] = fcn(KpGS, KiGS, KpKi, Scheduled)

if Scheduled > 0.5
    Kp_out = KpGS;
    Ki_out = KiGS;
else
    Kp_out = KpKi(1);
    Ki_out = KpKi(2);
end
